simulink model "QAM"  (R2021a)
settings: Solver=VariableStepAuto  StartTime=0.0  StopTime=10.0  RelTol=1e-3
libraries: commdigbbndam3 x6, commchan3 x3, commsink2 x3, dspquant2 x3, dspsrcs4 x2, dspsigops x1
settings Model: Creator=Bharat Gunhalkar  LastModifiedBy=Bharat Gunhalkar

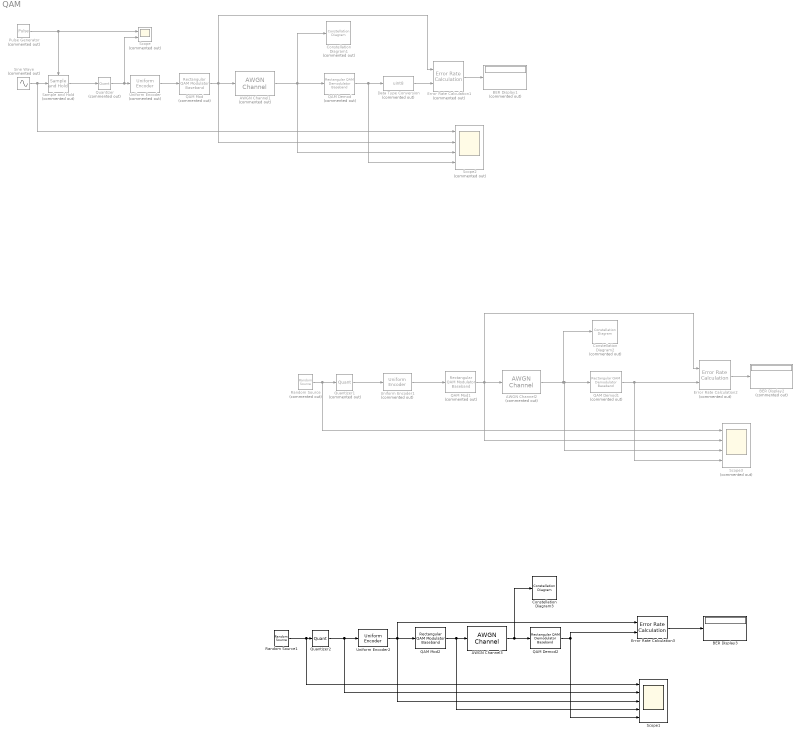
== system QAM ==
  AWGN Channel1 : commchan3/AWGN Channel  Commented=on  InputProcessing=Columns as channels (frame based)  seed=67  noiseMode="Signal to noise ratio  (Eb/No)"  EbNodB=1  EsNodB=10  SNRdB=10  bitsPerSym=1  Ps=1  Tsym=1  variance=1
  AWGN Channel2 : commchan3/AWGN Channel  Commented=on  InputProcessing=Columns as channels (frame based)  seed=67  noiseMode="Signal to noise ratio  (Eb/No)"  EbNodB=1  EsNodB=10  SNRdB=10  bitsPerSym=1  Ps=1  Tsym=1  variance=1
  AWGN Channel3 : commchan3/AWGN Channel  InputProcessing=Columns as channels (frame based)  seed=67  noiseMode="Signal to noise ratio  (Eb/No)"  EbNodB=1  EsNodB=10  SNRdB=10  bitsPerSym=1  Ps=1  Tsym=1  variance=1
  BER Display1 : Display  Commented=on
  BER Display2 : Display  Commented=on
  BER Display3 : Display
  Constellation Diagram1 : ConstellationDiagram  Commented=on
  Constellation Diagram2 : ConstellationDiagram  Commented=on
  Constellation Diagram3 : ConstellationDiagram
  Data Type Conversion : DataTypeConversion  Commented=on  OutDataTypeStr=uint8
  Error Rate Calculation1 : commsink2/Error Rate Calculation  Commented=on  N=0  st_delay=0  cp_mode=Entire frame  subframe=[]  PMode=Port  WsName=ErrorVec  RsMode2=off  stop=off  numErr=100  maxBits=1e6
  Error Rate Calculation2 : commsink2/Error Rate Calculation  Commented=on  N=0  st_delay=0  cp_mode=Entire frame  subframe=[]  PMode=Port  WsName=ErrorVec  RsMode2=off  stop=off  numErr=100  maxBits=1e6
  Error Rate Calculation3 : commsink2/Error Rate Calculation  N=0  st_delay=0  cp_mode=Entire frame  subframe=[]  PMode=Port  WsName=ErrorVec  RsMode2=off  stop=off  numErr=100  maxBits=1e6
  Pulse Generator : DiscretePulseGenerator  Commented=on  Period=1000  PulseWidth=5
  QAM Demod : commdigbbndam3/Rectangular QAM Demodulator Baseband  Commented=on  M=16  OutType=Integer  DecType=Hard decision  VarSource=Dialog  Variance=1  Dec=Gray  Mapping=[0:15]  PowType=Min. distance between symbols  MinDist=2  AvgPow=1  PeakPow=1  Ph=0  outDtype1=Inherit via internal rule  outDtype2=Inherit via internal rule  derotateFactorWordLen=16  derotateFactorDataTypeStr=Inherit: Same word length as input  derotateFactorLastDataTypeStr=Inherit: Same word length as input  denormFactorWordLen=16  denormFactorDataTypeStr=Inherit: Same word length as input  denormFactorLastDataTypeStr=Inherit: Same word length as input  prodOutWordLen=32  prodOutOverflowMode=Wrap  prodOutRoundingMode=Floor  prodOutOvFlMode=off  prodOutOvFlModeLastStrValue=off  sumWordLen=32
  QAM Demod1 : commdigbbndam3/Rectangular QAM Demodulator Baseband  Commented=on  M=16  OutType=Integer  DecType=Hard decision  VarSource=Dialog  Variance=1  Dec=Gray  Mapping=[0:15]  PowType=Min. distance between symbols  MinDist=2  AvgPow=1  PeakPow=1  Ph=0  outDtype1=Inherit via internal rule  outDtype2=Inherit via internal rule  derotateFactorWordLen=16  derotateFactorDataTypeStr=Inherit: Same word length as input  derotateFactorLastDataTypeStr=Inherit: Same word length as input  denormFactorWordLen=16  denormFactorDataTypeStr=Inherit: Same word length as input  denormFactorLastDataTypeStr=Inherit: Same word length as input  prodOutWordLen=32  prodOutOverflowMode=Wrap  prodOutRoundingMode=Floor  prodOutOvFlMode=off  prodOutOvFlModeLastStrValue=off  sumWordLen=32
  QAM Demod2 : commdigbbndam3/Rectangular QAM Demodulator Baseband  M=16  OutType=Integer  DecType=Hard decision  VarSource=Dialog  Variance=1  Dec=Gray  Mapping=[0:15]  PowType=Min. distance between symbols  MinDist=2  AvgPow=1  PeakPow=1  Ph=0  outDtype1=Inherit via internal rule  outDtype2=Inherit via internal rule  derotateFactorWordLen=16  derotateFactorDataTypeStr=Inherit: Same word length as input  derotateFactorLastDataTypeStr=Inherit: Same word length as input  denormFactorWordLen=16  denormFactorDataTypeStr=Inherit: Same word length as input  denormFactorLastDataTypeStr=Inherit: Same word length as input  prodOutWordLen=32  prodOutOverflowMode=Wrap  prodOutRoundingMode=Floor  prodOutOvFlMode=off  prodOutOvFlModeLastStrValue=off  sumWordLen=32
  QAM Mod : commdigbbndam3/Rectangular QAM Modulator Baseband  Commented=on  M=16  InType=Integer  Enc=Gray  Mapping=[0:15]  PowType=Min. distance between symbols  MinDist=2  AvgPow=1  PeakPow=1  Ph=0  outDtype=double  outWordLen=16  outUDDataType=sfix(16)  outFracLenMode=Best precision  outFracLen=15  outDataTypeStr=double  outLastDataTypeStr=double
  QAM Mod1 : commdigbbndam3/Rectangular QAM Modulator Baseband  Commented=on  M=16  InType=Integer  Enc=Gray  Mapping=[0:15]  PowType=Min. distance between symbols  MinDist=2  AvgPow=1  PeakPow=1  Ph=0  outDtype=double  outWordLen=16  outUDDataType=sfix(16)  outFracLenMode=Best precision  outFracLen=15  outDataTypeStr=double  outLastDataTypeStr=double
  QAM Mod2 : commdigbbndam3/Rectangular QAM Modulator Baseband  M=16  InType=Integer  Enc=Gray  Mapping=[0:15]  PowType=Min. distance between symbols  MinDist=2  AvgPow=1  PeakPow=1  Ph=0  outDtype=double  outWordLen=16  outUDDataType=sfix(16)  outFracLenMode=Best precision  outFracLen=15  outDataTypeStr=double  outLastDataTypeStr=double
  Quantizer : Quantizer  Commented=on  QuantizationInterval=0.25  LinearizeAsGain=off
  Quantizer1 : Quantizer  Commented=on  QuantizationInterval=0.25  LinearizeAsGain=off
  Quantizer2 : Quantizer  QuantizationInterval=0.25  LinearizeAsGain=off
  Random Source : dspsrcs4/Random Source  Commented=on  SrcType=Uniform  NormMethod=Ziggurat  CltLength=12  MinVal=0  MaxVal=1  MeanVal=0  VarVal=1  RepMode=Not repeatable  rawSeed=1  IsInherit=off  SampMode=Discrete  SampTime=0.1  SampFrame=1  DataType=Single  OutComplex=Real  OutputFrames=off
  Random Source1 : dspsrcs4/Random Source  SrcType=Uniform  NormMethod=Ziggurat  CltLength=12  MinVal=0  MaxVal=1  MeanVal=0  VarVal=1  RepMode=Not repeatable  rawSeed=1  IsInherit=off  SampMode=Discrete  SampTime=0.1  SampFrame=1  DataType=Single  OutComplex=Real  OutputFrames=off
  Sample and Hold : dspsigops/Sample and Hold  Commented=on  trig=Rising edge  initCond=0  latchinput=off
  Scope : Scope  Commented=on  NumInputPorts=2
  Scope1 : Scope  NumInputPorts=5
  Scope2 : Scope  Commented=on  NumInputPorts=4
  Scope3 : Scope  Commented=on  NumInputPorts=4
  Sine Wave : Sin  Commented=on  Amplitude=10  SampleTime=0
  Uniform Encoder : dspquant2/Uniform Encoder  Commented=on  peak=1  bits=4  otype=Unsigned integer
  Uniform Encoder1 : dspquant2/Uniform Encoder  Commented=on  peak=1  bits=4  otype=Unsigned integer
  Uniform Encoder2 : dspquant2/Uniform Encoder  peak=1  bits=4  otype=Unsigned integer
  wires:
  Uniform Encoder/1 -> QAM Mod/1
  Data Type Conversion/1 -> Error Rate Calculation1/2
  Quantizer/1 -> Scope/2, Uniform Encoder/1
  Pulse Generator/1 -> Sample and Hold/Trigger, Scope/1
  Sample and Hold/1 -> Quantizer/1
  QAM Mod/1 -> Scope2/2, Error Rate Calculation1/1, AWGN Channel1/1
  Sine Wave/1 -> Scope2/1, Sample and Hold/1
  AWGN Channel1/1 -> Scope2/3, QAM Demod/1, Constellation Diagram1/1
  QAM Demod/1 -> Scope2/4, Data Type Conversion/1
  Error Rate Calculation1/1 -> BER Display1/1
  Error Rate Calculation2/1 -> BER Display2/1
  AWGN Channel2/1 -> Scope3/3, QAM Demod1/1, Constellation Diagram2/1
  QAM Mod1/1 -> Scope3/2, Error Rate Calculation2/1, AWGN Channel2/1
  QAM Demod1/1 -> Error Rate Calculation2/2, Scope3/4
  Uniform Encoder1/1 -> QAM Mod1/1
  Random Source/1 -> Scope3/1, Quantizer1/1
  Quantizer1/1 -> Uniform Encoder1/1
  QAM Demod2/1 -> Error Rate Calculation3/2, Scope1/5
  Random Source1/1 -> Scope1/1, Quantizer2/1
  Error Rate Calculation3/1 -> BER Display3/1
  Quantizer2/1 -> Uniform Encoder2/1, Scope1/2
  Uniform Encoder2/1 -> QAM Mod2/1, Error Rate Calculation3/1, Scope1/3
  AWGN Channel3/1 -> QAM Demod2/1, Constellation Diagram3/1
  QAM Mod2/1 -> AWGN Channel3/1, Scope1/4
